simulink model "Question9Hw1_AkankshaMurali"  (R2023b)
settings: Solver=VariableStepAuto  StartTime=0.0  StopTime=10.0  RelTol=1e-3
settings Model: Creator=akank  LastModifiedBy=akank

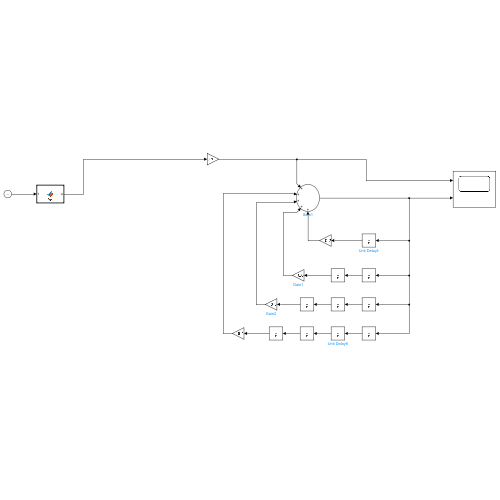
[thumbnail: Simulink's stored preview of the top-level diagram]
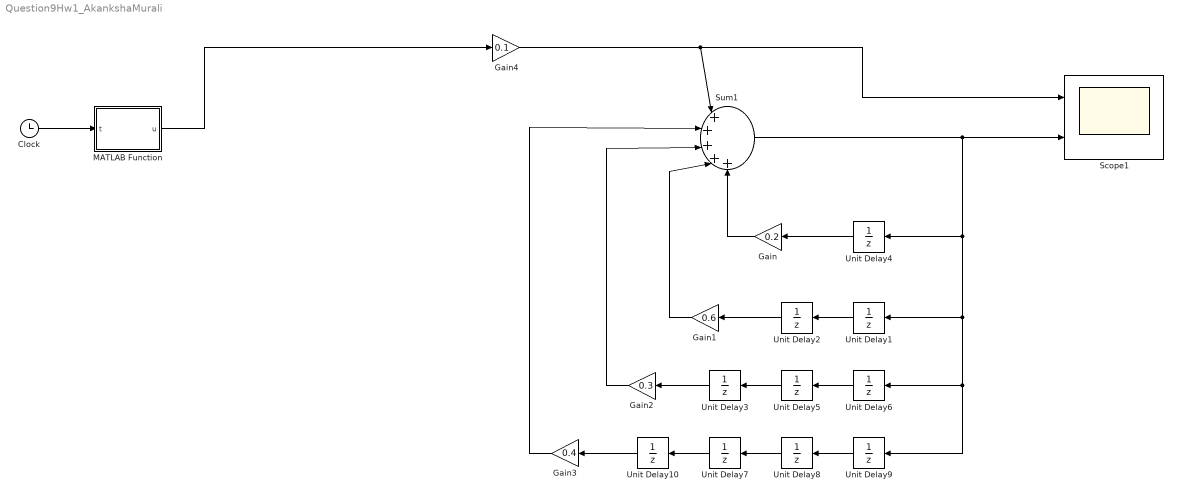
== system Question9Hw1_AkankshaMurali ==
  Clock : Clock
      settings: Decimation=4
  Gain : Gain  Gain=0.2
  Gain1 : Gain  Gain=0.6
  Gain2 : Gain  Gain=0.3
  Gain3 : Gain  Gain=0.4
  Gain4 : Gain  Gain=0.1
  MATLAB Function : MATLAB Function  TreatAsAtomicUnit=on
  Scope1 : Scope  NumInputPorts=2
  Sum1 : Sum  Inputs=|+++++
  Unit Delay{1..10} (10 alike) : UnitDelay  SampleTime=-1  HasFrameUpgradeWarning=on
  wires:
  MATLAB Function/1(u) -> Gain4/1
  Clock/1 -> MATLAB Function/1(t)
  Gain4/1 -> Sum1/1, Scope1/1
  Unit Delay5/1 -> Unit Delay3/1
  Unit Delay8/1 -> Unit Delay7/1
  Gain3/1 -> Sum1/2
  Gain2/1 -> Sum1/3
  Gain1/1 -> Sum1/4
  Gain/1 -> Sum1/5
  Sum1/1 -> Unit Delay4/1, Unit Delay1/1, Unit Delay6/1, Unit Delay9/1, Scope1/2
  Unit Delay4/1 -> Gain/1
  Unit Delay1/1 -> Unit Delay2/1
  Unit Delay2/1 -> Gain1/1
  Unit Delay6/1 -> Unit Delay5/1
  Unit Delay3/1 -> Gain2/1
  Unit Delay10/1 -> Gain3/1
  Unit Delay7/1 -> Unit Delay10/1
  Unit Delay9/1 -> Unit Delay8/1

== matlab function Question9Hw1_AkankshaMurali/MATLAB Function ==
  data: t input; u output
function u = fcn(t)

u = sin(t) + sin(2*t)+ sin(30*t) + sin(40*t);
